simulink model "dynamics_w_environment_model"  (R2022a)
settings: Solver=FixedStepAuto  StartTime=0.0  StopTime=3600  FixedStep=0.1  MaxStep=1  MinStep=0.01  RelTol=1e-3
undefined symbols (not defined in the file): km, s, WMM2020
libraries: aerolibutil x3, matrix_library x2, aerolibgravity2 x1, vrlib x1, aerolibcelestial x1
settings Model: SimulationMode=accelerator  Creator=samuel  LastModifiedBy=samuel

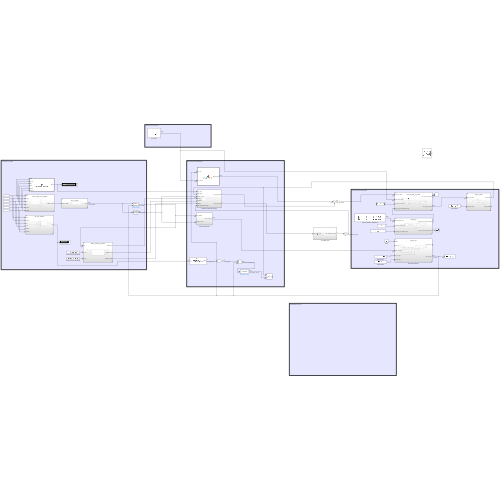
[thumbnail: Simulink's stored preview of the top-level diagram]
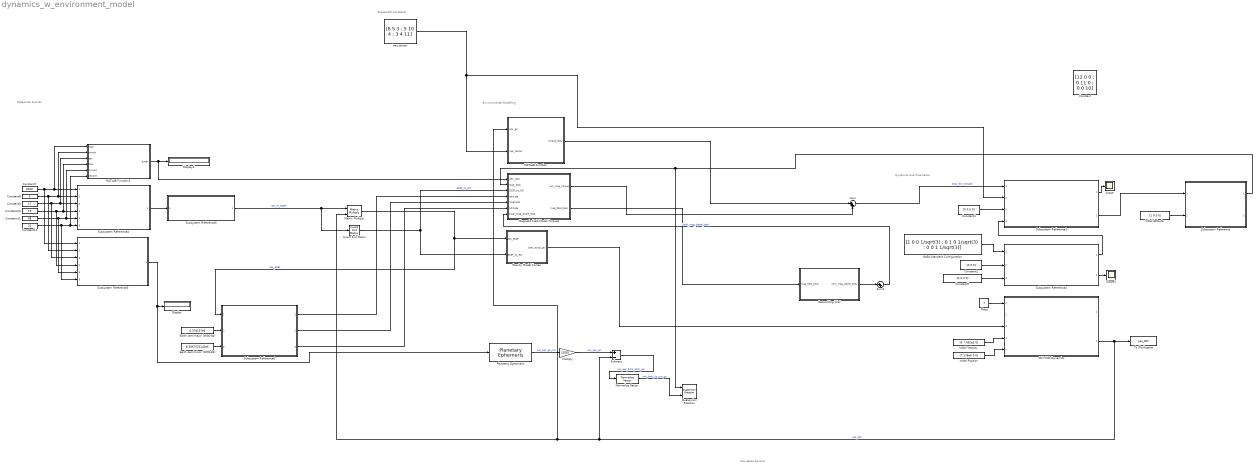
== system dynamics_w_environment_model ==
  note: Simulated Sensors
  note: Spacecraft Constants
  note: Reference Frames
  note: Environmental Modelling
  note: Dynamics and Kinematics
  Constant : Constant  Value=[12 0 0 ; 0 11 0 ; 0 0 10]
  Constant10 : Constant  Value=19
  Constant11 : Constant  Value=48
  Constant12 : Constant  Value=32
  Constant2 : Constant  Value=[0 0 0]
  Constant4 : Constant  Value=[0 0.5 0]
  Constant5 : Constant  Value=[0 0 0 0]
  Constant7 : Constant  Value=2020
  Constant8 : Constant  Value=3
  Constant9 : Constant  Value=17
  Detumbling Trial : Subsystem
  Display : Display
  Display4 : Display
  Earth semimajor (WGS-84) : Constant  Value=6.378137e6
  Earth semiminor (WGS-84) : Constant  Value=6.3567523142e6
  GCI COG Dynamics : Subsystem  ReferencedSubsystem=cog_dyn_gci
  Gravity Model Forces : Subsystem
  Initial Attitude : Constant  Value=[1 0 0 0]
  Initial Position : Constant  Value=[7.178e6 0 0]
  Initial Velocity : Constant  Value=[0 7.452e3 0]
  Invert 3x3 Matrix : aerolibutil/Invert  3x3 Matrix
  MATLAB Function : MATLAB Function  TreatAsAtomicUnit=on
  MATLAB Function1 : MATLAB Function  TreatAsAtomicUnit=on
  Magnetic Field Model Torques : Subsystem
  Mass : Constant  Value=7
  Matrix Multiply : Product  Multiplication=Matrix(*)
  Multiply : Gain  Gain=1000
  NASA Standard Configuration : Constant  Value=[1 0 0 1/sqrt(3) ; 0 1 0 1/sqrt(3) ; 0 0 1 1/sqrt(3)]
  Normalize Vector : vrlib/Utilities/Normalize Vector  maxzero=0
  Planetary Ephemeris : aerolibcelestial/Planetary Ephemeris  kmflag=km,km/s  epochflag=Julian date  de=DE405  nCenter=Earth  nTarget=Moon  errorflag=Error  velflag=off
      settings: SourceProductBaseCode=AE
  Quaternion Rotation : aerolibutil/Quaternion Rotation
  Scope : Scope
  Scope1 : Scope
  Subsystem Reference : Subsystem  ReferencedSubsystem=quat_kin_body
  Subsystem Reference1 : Subsystem  ReferencedSubsystem=quat_dyn_body_w_wheels
  Subsystem Reference2 : Subsystem  ReferencedSubsystem=wheel_dyn
  Subsystem Reference3 : Subsystem  ReferencedSubsystem=JD_from_datetime
  Subsystem Reference4 : Subsystem  ReferencedSubsystem=GMST_angle_from_datetime
  Subsystem Reference5 : Subsystem  ReferencedSubsystem=GCI_to_ECEF
  Subsystem Reference6 : Subsystem  ReferencedSubsystem=ECEF_coords_to_geodetic
  Subtract : Sum  Inputs=+-
  Sum : Sum  Inputs=|++
  Sum1 : Sum  Inputs=|++
  To Workspace : ToWorkspace  VariableName=pos_GCI  SampleTime=-1
  iner_tensor : Constant  Value=[8 5 3 ; 5 10 4 ; 3 4 11]
  wires:
  Subsystem Reference1/2 -> Subsystem Reference/1
  NASA Standard Configuration/1 -> Subsystem Reference2/1
  iner_tensor/1 -> Subsystem Reference1/2, MATLAB Function/2(iner_tensor)
  Subsystem Reference2/1 -> Subsystem Reference1/4
  Initial Attitude/1 -> Subsystem Reference/2
  Constant4/1 -> Subsystem Reference1/3
  Constant5/1 -> Subsystem Reference2/3
  Mass/1 -> GCI COG Dynamics/1
  Constant7/1 -> Subsystem Reference3/1, MATLAB Function1/1(year), Subsystem Reference4/1
  Constant8/1 -> Subsystem Reference3/2, MATLAB Function1/2(month), Subsystem Reference4/2
  Constant9/1 -> Subsystem Reference3/3, MATLAB Function1/3(day), Subsystem Reference4/3
  Constant10/1 -> Subsystem Reference3/4, MATLAB Function1/4(hour), Subsystem Reference4/4
  Constant11/1 -> Subsystem Reference3/5, MATLAB Function1/5(minute), Subsystem Reference4/5
  Constant12/1 -> Subsystem Reference3/6, MATLAB Function1/6(second), Subsystem Reference4/6
  Subsystem Reference4/1 -> Subsystem Reference5/1
  Subsystem Reference5/1 -> Matrix Multiply/1, Invert 3x3 Matrix/1  "GCI_to_ECEF"
  Matrix Multiply/1 -> Subsystem Reference6/1, Gravity Model Forces/1(pos_ECEF)  "pos_ECEF"
  Invert 3x3 Matrix/1 -> Magnetic Field Model Torques/3(ECEF_to_GCI), Gravity Model Forces/2(ECEF_to_GCI)  "ECEF_to_GCI"
  Initial Velocity/1 -> GCI COG Dynamics/4
  Initial Position/1 -> GCI COG Dynamics/5
  Sum/1 -> Subsystem Reference1/1  "total_ext_torques"
  MATLAB Function/1(torque_body) -> Sum/1
  Earth semimajor (WGS-84)/1 -> Subsystem Reference6/2
  Earth semiminor (WGS-84)/1 -> Subsystem Reference6/3
  GCI COG Dynamics/2 -> Subtract/2, MATLAB Function/1(pos_gci), Matrix Multiply/2, To Workspace/1  "pos_GCI"
  MATLAB Function1/1(dyear) -> Magnetic Field Model Torques/1(dec_year), Display4/1
  Constant2/1 -> Subsystem Reference2/2
  Subsystem Reference1/1 -> Scope/1
  Subsystem Reference2/2 -> Scope1/1
  Subsystem Reference3/1 -> Display/1, Planetary Ephemeris/1
  Planetary Ephemeris/1 -> Multiply/1  "sun_pos_gci_km"
  Detumbling Trial/1(com_mag_dipole_body) -> Sum1/1
  Subsystem Reference6/1 -> Magnetic Field Model Torques/4(latitude)
  Subsystem Reference6/2 -> Magnetic Field Model Torques/5(longitude)
  Subsystem Reference6/3 -> Magnetic Field Model Torques/6(altitude)
  Sum1/1 -> Magnetic Field Model Torques/7(total_mag_dipole_body)  "total_mag_dipole_body"
  Magnetic Field Model Torques/1(ext_mag_torque) -> Sum/2
  Magnetic Field Model Torques/2(mag_field_body) -> Detumbling Trial/1(mag_field_body)
  Gravity Model Forces/1(grav_accel_gci) -> GCI COG Dynamics/3
  Subtract/1 -> Normalize Vector/1  "sun_pos_from_body_gci"
  Multiply/1 -> Subtract/1  "sun_pos_gci"
  Normalize Vector/1 -> Quaternion Rotation/2  "unit_body_to_sun_gci"
  Subsystem Reference/1 -> Quaternion Rotation/1, Magnetic Field Model Torques/2(quat_body)

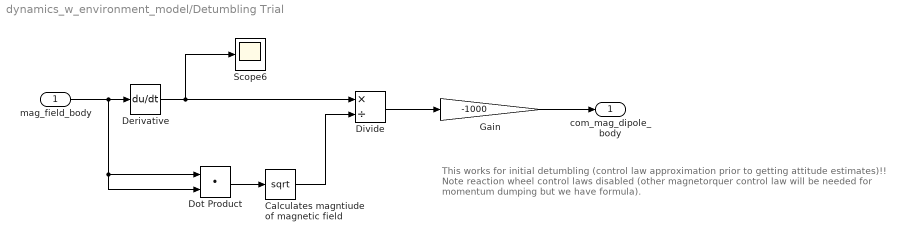
== system dynamics_w_environment_model/Detumbling Trial ==
  note: This works for initial detumbling (control law approximation prior to getting attitude estimates)!! Note reaction wheel control laws disabled (other magnetorquer control law will be needed for momentum dumping but we have formula).
  mag_field_body : Inport
  Calculates magntiude of magnetic field : Sqrt
  Derivative : Derivative
  Divide : Product  Inputs=*/
  Dot Product : DotProduct  OutDataTypeStr=Inherit: Inherit via internal rule
  Gain : Gain  Gain=-1000
  Scope6 : Scope
  com_mag_dipole_body : Outport
  wires:
  Calculates magntiude of magnetic field/1 -> Divide/2
  Gain/1 -> com_mag_dipole_body/1
  Dot Product/1 -> Calculates magntiude of magnetic field/1
  Divide/1 -> Gain/1
  mag_field_body/1 -> Derivative/1, Dot Product/2, Dot Product/1
  Derivative/1 -> Divide/1, Scope6/1

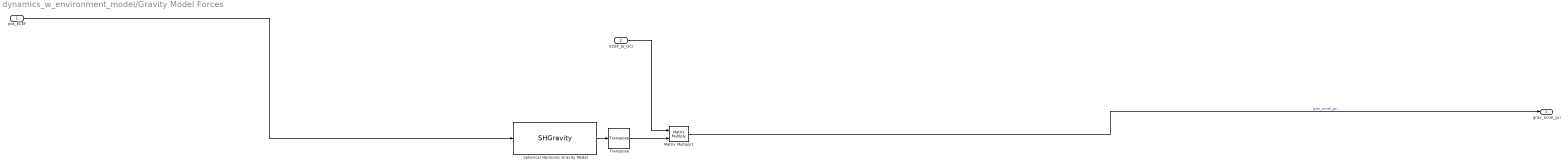
== system dynamics_w_environment_model/Gravity Model Forces ==
  pos_ECEF : Inport
  ECEF_to_GCI : Inport  Port=2
  Matrix Multiply1 : Product  Multiplication=Matrix(*)
  Spherical Harmonic Gravity Model : SHGravity
  Transpose : matrix_library/Transpose
      settings: SourceProductBaseCode=SL
  grav_accel_gci : Outport
  wires:
  Spherical Harmonic Gravity Model/1 -> Transpose/1
  Transpose/1 -> Matrix Multiply1/2
  ECEF_to_GCI/1 -> Matrix Multiply1/1
  pos_ECEF/1 -> Spherical Harmonic Gravity Model/1
  Matrix Multiply1/1 -> grav_accel_gci/1  "grav_accel_gci"

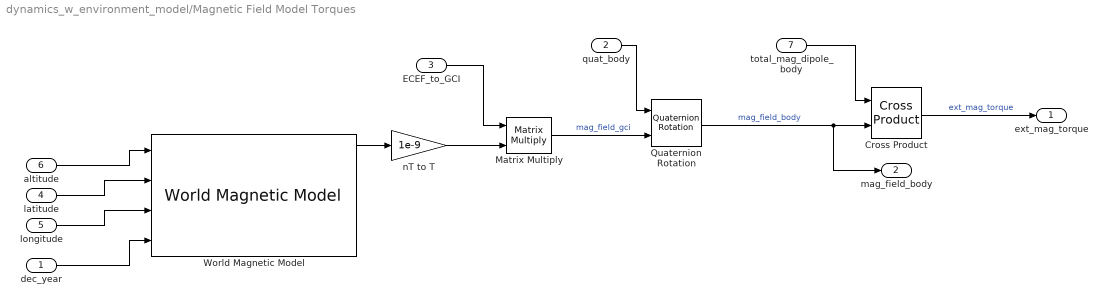
== system dynamics_w_environment_model/Magnetic Field Model Torques ==
  dec_year : Inport
  quat_body : Inport  Port=2
  ECEF_to_GCI : Inport  Port=3
  latitude : Inport  Port=4
  longitude : Inport  Port=5
  altitude : Inport  Port=6
  total_mag_dipole_body : Inport  Port=7
  Cross Product : matrix_library/Cross Product
      settings: SourceProductBaseCode=SL
  Matrix Multiply : Product  Multiplication=Matrix(*)
  Quaternion Rotation : aerolibutil/Quaternion Rotation
  World Magnetic Model : aerolibgravity2/World Magnetic Model  model=WMM2020 (2020-2025)  customFile='WMM2020.COF'  units=Metric (MKS)  time_in=on  month=January  day=1  year=2020  action=Error  h_out=on  dec_out=on  inc_out=on  ti_out=on
      settings: SourceProductBaseCode=AE
  nT to T : Gain  Gain=1e-9
  ext_mag_torque : Outport
  mag_field_body : Outport  Port=2
  wires:
  latitude/1 -> World Magnetic Model/2
  quat_body/1 -> Quaternion Rotation/1
  altitude/1 -> World Magnetic Model/1
  World Magnetic Model/1 -> nT to T/1
  total_mag_dipole_body/1 -> Cross Product/1
  Matrix Multiply/1 -> Quaternion Rotation/2  "mag_field_gci"
  Cross Product/1 -> ext_mag_torque/1  "ext_mag_torque"
  Quaternion Rotation/1 -> mag_field_body/1, Cross Product/2  "mag_field_body"
  nT to T/1 -> Matrix Multiply/2
  ECEF_to_GCI/1 -> Matrix Multiply/1
  longitude/1 -> World Magnetic Model/3
  dec_year/1 -> World Magnetic Model/4

== matlab function dynamics_w_environment_model/MATLAB Function ==
  data: pos_gci input; torque_body output; iner_tensor input
function torque_body  = grav_grad_torque(pos_gci, iner_tensor)
    % mass of earth, grav constant
    m_e = 5.97219e24;
    G = 6.67430e-11;

    % grav param
    u = G*m_e;

    radius = norm(pos_gci);
    nadir_vec = -normalize(pos_gci);
    torque_body = cross(3*u/radius^3*nadir_vec, ...
        iner_tensor*nadir_vec);

== matlab function dynamics_w_environment_model/MATLAB Function1 ==
  data: year input; dyear output; month input; day input; hour input; minute input; second input
function dyear = dyear_from_datetime(year, month, day, hour, minute, second)
    % sequentially builds the decimal year
    tot_mins = minute + second/60; % use 61 for leap second days? probably fine
    tot_hours = hour + tot_mins / 60;
    tot_days = day + tot_hours / 24;
    tot_months = month + tot_days / (275/9); % average days in month across year
    tot_years = year + tot_months / 12;

    dyear = tot_years;
